simulink model "TestModel"  (R2018a)
settings: Solver=ode1  StartTime=0.0  StopTime=inf  FixedStep=T  RelTol=1e-3  EnableMultiTasking=on
undefined symbols (not defined in the file): DiscIntNeverNeededParam, host, port, T
libraries: simulink x3
settings Model: PacingRate=1.200000  Creator=AMM  LastModifiedBy=AMM
settings SolverCC: ZeroCrossControl=DisableAll
settings HardwareCC: TargetBitPerPointer=64  TargetBitPerSizeT=64  TargetBitPerPtrDiffT=64  TargetLongLongMode=on  TargetIntDivRoundTo=Zero  TargetEndianess=LittleEndian  TargetWordSize=64  TargetHWDeviceType=MATLAB Host  ProdEqTarget=off
settings RTWCC: SystemTargetFile=rsim.tlc  TemplateMakefile=rsim_default_tmf  Description=Rapid Simulation Target  BuildConfiguration=Faster Runs  TargetLang=C++  RTWCompilerOptimization=on
settings RSimTargetCC: TargetLangStandard=C++03 (ISO)  GeneratePreprocessorConditionals=Use local settings

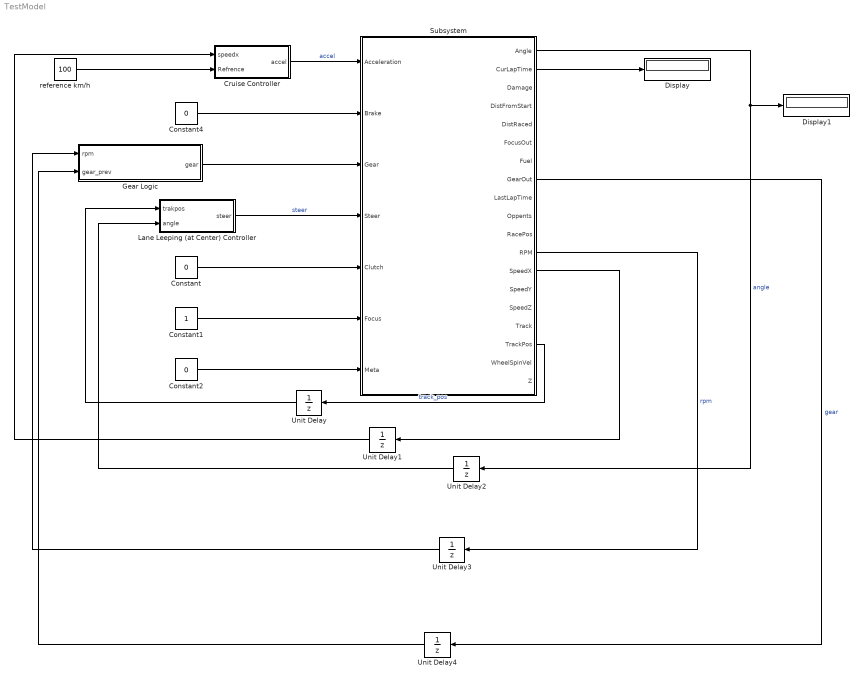
== system TestModel ==
  Constant : Constant  Value=0
  Constant1 : Constant
  Constant2 : Constant  Value=0
  Constant4 : Constant  Value=0
  Cruise Controller : Subsystem  Priority=0
  Display : Display
  Display1 : Display
  Gear Logic : MATLAB Function  TreatAsAtomicUnit=on
  Lane Leeping (at Center) Controller : Subsystem  Priority=0
  Subsystem : Subsystem  Priority=1
  Unit Delay{,1..3} (4 alike) : UnitDelay  SampleTime=-1
  Unit Delay4 : UnitDelay  InitialCondition=1  SampleTime=-1
  reference km/h : Constant  Value=100
  wires:
  Lane Leeping (at Center) Controller/1(steer) -> Subsystem/4(Steer)  "steer"
  Constant/1 -> Subsystem/5(Clutch)
  Constant1/1 -> Subsystem/6(Focus)
  Constant2/1 -> Subsystem/7(Meta)
  Constant4/1 -> Subsystem/2(Brake)
  Subsystem/13(SpeedX) -> Unit Delay1/1
  Cruise Controller/1(accel) -> Subsystem/1(Acceleration)  "accel"
  Subsystem/17(TrackPos) -> Unit Delay/1  "track_pos"
  Subsystem/1(Angle) -> Display1/1, Unit Delay2/1  "angle"
  reference km/h/1 -> Cruise Controller/2("Refrence ")
  Unit Delay/1 -> Lane Leeping (at Center) Controller/1(trakpos)
  Unit Delay1/1 -> Cruise Controller/1("speedx ")
  Unit Delay2/1 -> Lane Leeping (at Center) Controller/2(angle)
  Subsystem/2(CurLapTime) -> Display/1
  Gear Logic/1(gear) -> Subsystem/3(Gear)
  Subsystem/12(RPM) -> Unit Delay3/1  "rpm"
  Subsystem/8(GearOut) -> Unit Delay4/1  "gear"
  Unit Delay3/1 -> Gear Logic/1(rpm)
  Unit Delay4/1 -> Gear Logic/2(gear_prev)

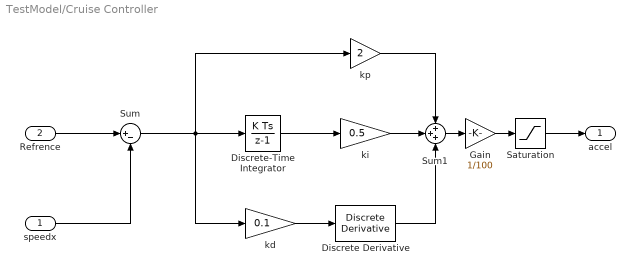
== system TestModel/Cruise Controller ==
  "speedx " : Inport
  "Refrence " : Inport  Port=2
  Discrete Derivative : simulink/Discrete/Discrete Derivative  gainval=1.0  ICPrevScaledInput=0.0  OutMin=[]  OutMax=[]  OutDataType=fixdt(1, 16)  OutScaling=2^-10  DoSatur=off
  Discrete-Time Integrator : DiscreteIntegrator  SampleTime=-1  ICPrevOutput=DiscIntNeverNeededParam  ICPrevScaledInput=DiscIntNeverNeededParam
  Gain : Gain  Gain=1/100
  Saturation : Saturate  UpperLimit=1  LowerLimit=-1
  Sum : Sum  Inputs=|+-
  Sum1 : Sum  Inputs=+++
  "kd " : Gain  Gain=0.1
  "ki " : Gain  Gain=0.5
  kp : Gain  Gain=2
  accel : Outport
  wires:
  "speedx "/1 -> Sum/2
  "Refrence "/1 -> Sum/1
  Sum/1 -> Discrete-Time Integrator/1, "kd "/1, kp/1
  "kd "/1 -> Discrete Derivative/1
  kp/1 -> Sum1/1
  Sum1/1 -> Gain/1
  Saturation/1 -> accel/1
  Gain/1 -> Saturation/1
  "ki "/1 -> Sum1/2
  Discrete-Time Integrator/1 -> "ki "/1
  Discrete Derivative/1 -> Sum1/3

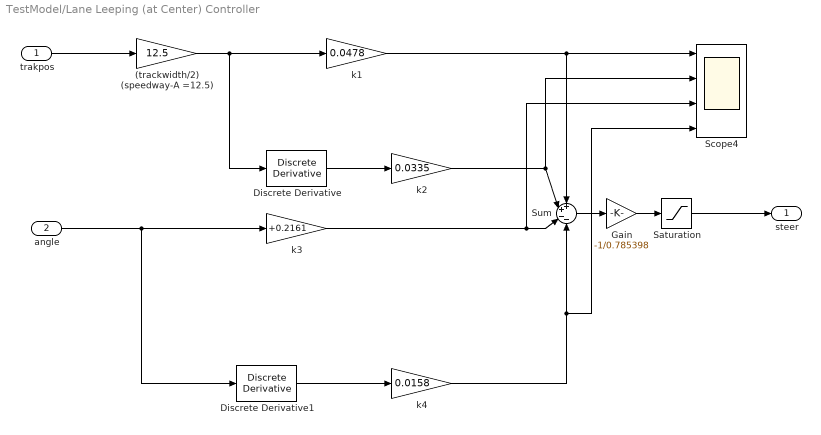
== system TestModel/Lane Leeping (at Center) Controller ==
  trakpos : Inport
  angle : Inport  Port=2
  (trackwidth/2) (speedway-A =12.5) : Gain  Gain=12.5
  Discrete Derivative : simulink/Discrete/Discrete Derivative  gainval=1.0  ICPrevScaledInput=0.0  OutMin=[]  OutMax=[]  OutDataType=fixdt(1, 16)  OutScaling=2^-10  DoSatur=off
  Discrete Derivative1 : simulink/Discrete/Discrete Derivative  gainval=1.0  ICPrevScaledInput=0.0  OutMin=[]  OutMax=[]  OutDataType=fixdt(1, 16)  OutScaling=2^-10  DoSatur=off
  Gain : Gain  Gain=-1/0.785398
  Saturation : Saturate  UpperLimit=1  LowerLimit=-1
  Scope4 : Scope  NumInputPorts=4
  Sum : Sum  Inputs=++--
  k1 : Gain  Gain=0.0478
  k2 : Gain  Gain=0.0335
  k3 : Gain  Gain=+0.2161
  k4 : Gain  Gain=0.0158
  steer : Outport
  wires:
  Sum/1 -> Gain/1
  angle/1 -> Discrete Derivative1/1, k3/1
  (trackwidth/2) (speedway-A =12.5)/1 -> Discrete Derivative/1, k1/1
  Gain/1 -> Saturation/1
  k1/1 -> Scope4/1, Sum/1
  k2/1 -> Sum/2, Scope4/2
  k3/1 -> Scope4/3, Sum/3
  trakpos/1 -> (trackwidth/2) (speedway-A =12.5)/1
  Saturation/1 -> steer/1
  k4/1 -> Scope4/4, Sum/4
  Discrete Derivative/1 -> k2/1
  Discrete Derivative1/1 -> k4/1

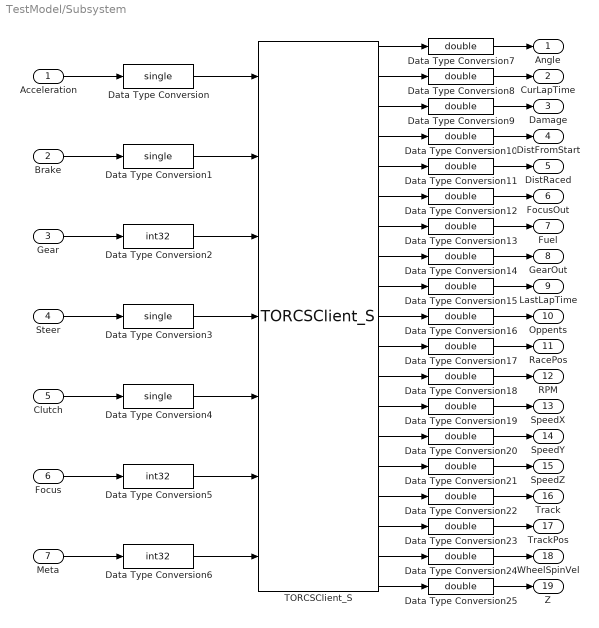
== system TestModel/Subsystem ==
  Acceleration : Inport
  Brake : Inport  Port=2
  Gear : Inport  Port=3
  Steer : Inport  Port=4
  Clutch : Inport  Port=5
  Focus : Inport  Port=6
  Meta : Inport  Port=7
  Data Type Conversion{,1,3..4} (4 alike) : DataTypeConversion  OutDataTypeStr=single
  Data Type Conversion{7..25} (19 alike) : DataTypeConversion  OutDataTypeStr=double
  Data Type Conversion2 : DataTypeConversion  OutDataTypeStr=int32
  Data Type Conversion5 : DataTypeConversion  OutDataTypeStr=int32
  Data Type Conversion6 : DataTypeConversion  OutDataTypeStr=int32
  TORCSClient_S : S-Function  FunctionName=TORCSClient_S  Parameters=host,port,T  SFunctionDeploymentMode=off  EnableBusSupport=off
  Angle : Outport
  CurLapTime : Outport  Port=2
  Damage : Outport  Port=3
  DistFromStart : Outport  Port=4
  DistRaced : Outport  Port=5
  FocusOut : Outport  Port=6
  Fuel : Outport  Port=7
  GearOut : Outport  Port=8
  LastLapTime : Outport  Port=9
  Oppents : Outport  Port=10
  RacePos : Outport  Port=11
  RPM : Outport  Port=12
  SpeedX : Outport  Port=13
  SpeedY : Outport  Port=14
  SpeedZ : Outport  Port=15
  Track : Outport  Port=16
  TrackPos : Outport  Port=17
  WheelSpinVel : Outport  Port=18
  Z : Outport  Port=19
  wires:
  Data Type Conversion18/1 -> RPM/1
  TORCSClient_S/18 -> Data Type Conversion24/1
  Data Type Conversion7/1 -> Angle/1
  Data Type Conversion10/1 -> DistFromStart/1
  Data Type Conversion22/1 -> Track/1
  TORCSClient_S/19 -> Data Type Conversion25/1
  Brake/1 -> Data Type Conversion1/1
  Data Type Conversion16/1 -> Oppents/1
  TORCSClient_S/13 -> Data Type Conversion19/1
  Data Type Conversion3/1 -> TORCSClient_S/4
  Data Type Conversion25/1 -> Z/1
  TORCSClient_S/3 -> Data Type Conversion9/1
  TORCSClient_S/8 -> Data Type Conversion14/1
  TORCSClient_S/9 -> Data Type Conversion15/1
  Clutch/1 -> Data Type Conversion4/1
  TORCSClient_S/4 -> Data Type Conversion10/1
  TORCSClient_S/6 -> Data Type Conversion12/1
  Data Type Conversion14/1 -> GearOut/1
  TORCSClient_S/2 -> Data Type Conversion8/1
  TORCSClient_S/10 -> Data Type Conversion16/1
  Data Type Conversion4/1 -> TORCSClient_S/5
  Data Type Conversion15/1 -> LastLapTime/1
  Data Type Conversion5/1 -> TORCSClient_S/6
  Data Type Conversion/1 -> TORCSClient_S/1
  TORCSClient_S/16 -> Data Type Conversion22/1
  TORCSClient_S/15 -> Data Type Conversion21/1
  Data Type Conversion2/1 -> TORCSClient_S/3
  Data Type Conversion19/1 -> SpeedX/1
  Data Type Conversion20/1 -> SpeedY/1
  Data Type Conversion1/1 -> TORCSClient_S/2
  TORCSClient_S/11 -> Data Type Conversion17/1
  Data Type Conversion23/1 -> TrackPos/1
  TORCSClient_S/12 -> Data Type Conversion18/1
  TORCSClient_S/14 -> Data Type Conversion20/1
  TORCSClient_S/7 -> Data Type Conversion13/1
  TORCSClient_S/5 -> Data Type Conversion11/1
  TORCSClient_S/1 -> Data Type Conversion7/1
  TORCSClient_S/17 -> Data Type Conversion23/1
  Gear/1 -> Data Type Conversion2/1
  Data Type Conversion6/1 -> TORCSClient_S/7
  Data Type Conversion9/1 -> Damage/1
  Data Type Conversion17/1 -> RacePos/1
  Data Type Conversion12/1 -> FocusOut/1
  Acceleration/1 -> Data Type Conversion/1
  Data Type Conversion21/1 -> SpeedZ/1
  Meta/1 -> Data Type Conversion6/1
  Data Type Conversion24/1 -> WheelSpinVel/1
  Data Type Conversion8/1 -> CurLapTime/1
  Focus/1 -> Data Type Conversion5/1
  Steer/1 -> Data Type Conversion3/1
  Data Type Conversion13/1 -> Fuel/1
  Data Type Conversion11/1 -> DistRaced/1

== matlab function TestModel/Gear Logic ==
  data: rpm input; gear output; gear_prev input
function gear = fcn(rpm, gear_prev)

gearUp=[5000,6000,6000,6500,7000,0];
gearDown=[0,2500,3000,3000,3500,3500];

if(gear_prev < 1)
    gear=1;
    return;
end;

if(gear_prev<6 && rpm>=gearUp(gear_prev))
    gear=gear_prev+1;
    return;
else
    if(gear_prev>1 && rpm<=gearDown(gear_prev))
        gear=gear_prev-1;
        return;
    else
        gear=gear_prev;
        return;
    end;
end;
